simulink model "LQG_non_linear"  (R2022b)
settings: Solver=VariableStepAuto  StartTime=0.0  StopTime=100  RelTol=1e-3
values from neighbouring files (symbols this model uses):
  a = Mv+mp+2*ma+2*IAy/(ra^2)    (= 19.1666666667)    [function_f.m]
  b = 1/2*(Mv*l^2+mp*L^2+2*ma*d^2+IGz+IPz+2*IAz+2*IAy*(d/ra)^2)    (= 3.3525)    [function_f.m]
  IPy = 0.15    [function_f.m]
  IPz = 0.23    [function_f.m]
  Kr = lqr(J.A,J.B,Q,R)    [LQG.m]    (also in LQG_integrator.m = lqr(A,B,Q,R); LQG_with_integrator.m = lqr(A,B,Q,R))
  L = 1    [function_f.m]
  rp = 0.3    [function_f.m]
undefined symbols (not defined in the file or in its folder): std_dev_dy, std_dev_phi_dot, std_dev_psi, std_dev_tau_phi, std_dev_tau_psi, std_dev_theta, X_start_lqg_nonlin
libraries: simulink x5, sharedTrackingLibrary x1
settings Model: Creator=alexi  LastModifiedBy=Giorgia

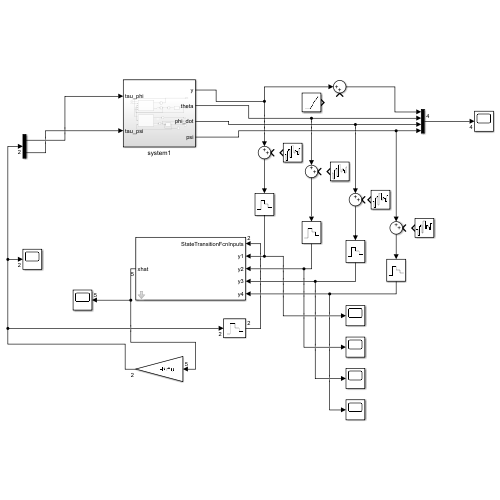
[thumbnail: Simulink's stored preview of the top-level diagram]
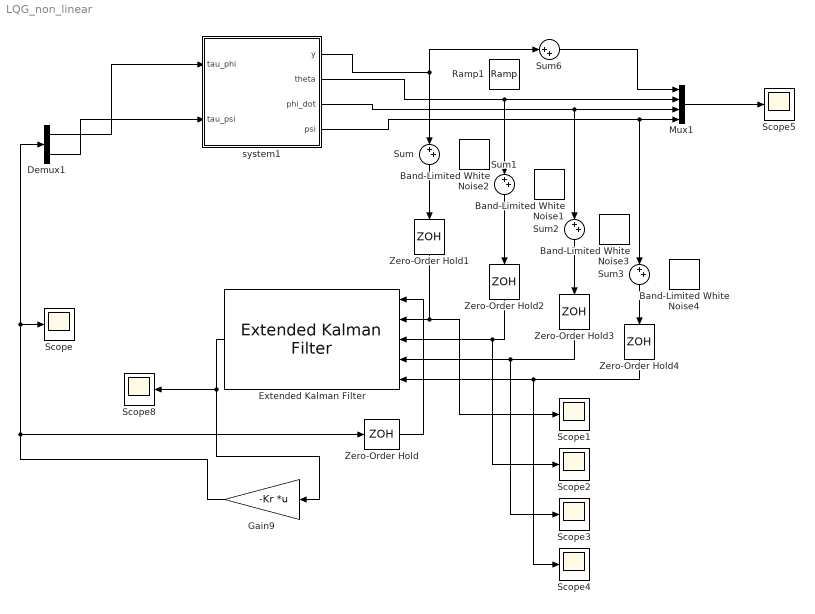
== system LQG_non_linear ==
  Band-Limited White Noise1 : simulink/Sources/Band-Limited White Noise  Cov=std_dev_theta^2  Ts=0.01  seed=[23341]
  Band-Limited White Noise2 : simulink/Sources/Band-Limited White Noise  Cov=std_dev_dy^2  Ts=0.01  seed=[23341]
  Band-Limited White Noise3 : simulink/Sources/Band-Limited White Noise  Cov=std_dev_phi_dot^2  Ts=0.01  seed=[23341]
  Band-Limited White Noise4 : simulink/Sources/Band-Limited White Noise  Cov=std_dev_psi^2  Ts=0.01  seed=[23341]
  Demux1 : Demux  Outputs=2
  Extended Kalman Filter : sharedTrackingLibrary/Extended Kalman Filter  StateTransitionFcn=function_f  HasStateTransitionJacobianFcn=off  HasAdditiveProcessNoise=Additive  ProcessNoise=[0 0 0 0 0; 0 0 0 0 0; 0 0 std_dev_tau_phi^2 0 0; 0 0 0 0 0; 0 0 0 0 std_dev_tau_psi^2]  HasTimeVaryingProcessNoise=off  HasStateTransitionFcnExtraArgument=1  InitialState=X_start_lqg_nonlin  InitialStateCovariance=1e-6  MeasurementFcn1=function_h1  HasMeasurementJacobianFcn1=off  HasMeasurementEnablePort1=off  HasAdditiveMeasurementNoise1=Additive  MeasurementNoise1=std_dev_dy^2  HasTimeVaryingMeasurementNoise1=off  HasMeasurementFcnExtraArgument1=0  HasMeasurementWrapping1=off  MeasurementFcn2=function_h2  HasMeasurementJacobianFcn2=off  HasMeasurementEnablePort2=off  HasAdditiveMeasurementNoise2=Additive  MeasurementNoise2=std_dev_theta^2  HasTimeVaryingMeasurementNoise2=off  HasMeasurementFcnExtraArgument2=0  HasMeasurementWrapping2=off  MeasurementFcn3=function_h3  HasMeasurementJacobianFcn3=off  HasMeasurementEnablePort3=off  HasAdditiveMeasurementNoise3=Additive  MeasurementNoise3=std_dev_phi_dot^2  HasTimeVaryingMeasurementNoise3=off  HasMeasurementFcnExtraArgument3=0  HasMeasurementWrapping3=off  MeasurementFcn4=function_h4  HasMeasurementJacobianFcn4=off  HasMeasurementEnablePort4=off  HasAdditiveMeasurementNoise4=Additive  MeasurementNoise4=std_dev_psi^2  HasTimeVaryingMeasurementNoise4=off  HasMeasurementFcnExtraArgument4=0  HasMeasurementWrapping4=off  MeasurementFcn5=myMeasurementFcn  HasMeasurementJacobianFcn5=off  HasMeasurementEnablePort5=off  HasAdditiveMeasurementNoise5=Additive  MeasurementNoise5=1  HasTimeVaryingMeasurementNoise5=off  HasMeasurementFcnExtraArgument5=0  HasMeasurementWrapping5=off  EnableMultirate=off  StateTransitionFcnSampleTime=1  MeasurementFcn1SampleTime=1  MeasurementFcn2SampleTime=1  MeasurementFcn3SampleTime=1  MeasurementFcn4SampleTime=1  MeasurementFcn5SampleTime=1  UseCurrentEstimator=on  OutputStateCovariance=off  DataType=double  SampleTime=0.01  NumberOfMeasurements=4
  Gain9 : Gain  Gain=-Kr  Multiplication=Matrix(K*u)
  Mux1 : Mux
  Ramp1 : simulink/Sources/Ramp  slope=1  start=0  InitialOutput=0
  Scope{,1..5,8} (7 alike) : Scope
  Sum{,1..3,6} (5 alike) : Sum  Inputs=|++
  Zero-Order Hold{,1..4} (5 alike) : ZeroOrderHold  SampleTime=0.01
  system1 : Subsystem
  wires:
  Mux1/1 -> Scope5/1
  Sum6/1 -> Mux1/1
  system1/2(theta) -> Sum1/1, Mux1/2
  system1/3(phi_dot) -> Sum2/1, Mux1/3
  system1/4(psi) -> Sum3/1, Mux1/4
  Demux1/1 -> system1/1(tau_phi)
  Demux1/2 -> system1/2(tau_psi)
  Gain9/1 -> Demux1/1, Scope/1, Zero-Order Hold/1
  Zero-Order Hold/1 -> Extended Kalman Filter/1
  system1/1(y) -> Sum6/1, Sum/1
  Extended Kalman Filter/1 -> Scope8/1, Gain9/1
  Zero-Order Hold1/1 -> Scope1/1, Extended Kalman Filter/2
  Zero-Order Hold2/1 -> Scope2/1, Extended Kalman Filter/3
  Zero-Order Hold3/1 -> Scope3/1, Extended Kalman Filter/4
  Zero-Order Hold4/1 -> Scope4/1, Extended Kalman Filter/5
  Sum/1 -> Zero-Order Hold1/1
  Sum1/1 -> Zero-Order Hold2/1
  Sum2/1 -> Zero-Order Hold3/1
  Sum3/1 -> Zero-Order Hold4/1

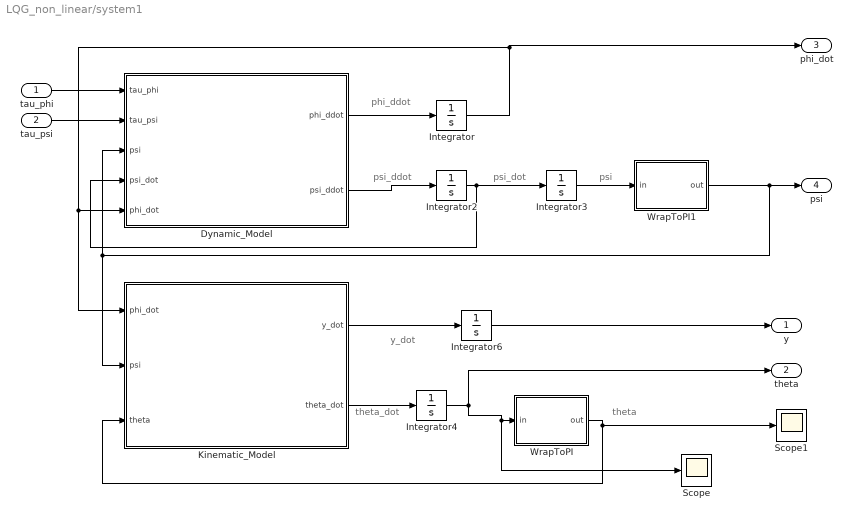
== system LQG_non_linear/system1 ==
  note: theta_dot
  note: psi_dot
  note: psi_ddot
  note: phi_ddot
  note: psi
  note: theta
  note: y_dot
  tau_phi : Inport
  tau_psi : Inport  Port=2
  Dynamic_Model : MATLAB Function  TreatAsAtomicUnit=on
  Integrator : Integrator  InitialCondition=X_start_lqg_nonlin(3)
  Integrator2 : Integrator  InitialCondition=X_start_lqg_nonlin(5)
  Integrator3 : Integrator  InitialCondition=X_start_lqg_nonlin(4)
  Integrator4 : Integrator  InitialCondition=X_start_lqg_nonlin(2)
  Integrator6 : Integrator  InitialCondition=X_start_lqg_nonlin(1)
  Kinematic_Model : MATLAB Function  TreatAsAtomicUnit=on
  Scope : Scope
  Scope1 : Scope
  WrapToPI : MATLAB Function  TreatAsAtomicUnit=on
  WrapToPI1 : MATLAB Function  TreatAsAtomicUnit=on
  y : Outport
  theta : Outport  Port=2
  phi_dot : Outport  Port=3
  psi : Outport  Port=4
  wires:
  Integrator6/1 -> y/1
  WrapToPI1/1(out) -> psi/1, Dynamic_Model/3(psi), Kinematic_Model/2(psi)
  Integrator2/1 -> Integrator3/1, Dynamic_Model/4(psi_dot)
  tau_phi/1 -> Dynamic_Model/1(tau_phi)
  Integrator3/1 -> WrapToPI1/1(in)
  Integrator4/1 -> Scope/1, WrapToPI/1(in), theta/1
  Integrator/1 -> Kinematic_Model/1(phi_dot), Dynamic_Model/5(phi_dot), phi_dot/1
  Kinematic_Model/1(y_dot) -> Integrator6/1
  Kinematic_Model/2(theta_dot) -> Integrator4/1
  Dynamic_Model/2(psi_ddot) -> Integrator2/1
  Dynamic_Model/1(phi_ddot) -> Integrator/1
  WrapToPI/1(out) -> Kinematic_Model/3(theta), Scope1/1
  tau_psi/1 -> Dynamic_Model/2(tau_psi)

== matlab function LQG_non_linear/system1/Dynamic_Model ==
  data: tau_phi input; tau_psi input; phi_ddot output; psi input; psi_dot input; phi_dot input; psi_ddot output; IPz parameter; IPy parameter; L parameter; rp parameter; b parameter; a parameter
function [phi_ddot,psi_ddot] = DynamicModel(tau_phi,tau_psi,psi,psi_dot,phi_dot,IPz, IPy, L, rp, b, a)
    B = [a*rp^2*cos(psi)^2+b*(rp/L)^2*sin(psi)^2+IPy, -IPz*(rp/L)*sin(psi)
        -IPz*(rp/L)*sin(psi), IPz];
    
    C = [(rp^2*b/L^2-a*rp^2)*cos(psi)*sin(psi)*psi_dot*phi_dot;
            -IPz*rp/L*cos(psi)*psi_dot*phi_dot];

    tau = [tau_phi;
            tau_psi];

    q_ddot = inv(B) * (tau - C);

    phi_ddot = q_ddot(1,:);
    psi_ddot = q_ddot(2,:);

== matlab function LQG_non_linear/system1/Kinematic_Model ==
  data: phi_dot input; psi input; theta input; y_dot output; theta_dot output; rp parameter; L parameter
function [y_dot,theta_dot] = KinematicModel(phi_dot,psi,theta,rp, L)
    x_dot = rp * phi_dot * cos(theta) * cos(psi);
    y_dot = rp * phi_dot * sin(theta) * cos(psi);
    theta_dot = - (rp * phi_dot * sin(psi)) / L;

== matlab function LQG_non_linear/system1/WrapToPI ==
  data: in input; out output
function out = wrapper(in)
    out = wrapTo2Pi(in);

== matlab function LQG_non_linear/system1/WrapToPI1 ==
  data: in input; out output
function out = wrapper(in)
    out = wrapToPi(in);
